simulink model "model_verification"  (R2024b)
settings: Solver=VariableStepAuto  StartTime=0.0  StopTime=10.0  RelTol=1e-3
undefined symbols (not defined in the file or in its folder): EulersEOM, IAU, juliandate, sat, WMM2020
libraries: aerolibutil x8, matrix_library x8, simulink_extras x6, sharedtransform x5, sharedutil x1, aerolibtransform2 x1, aerolibgravity2 x1
settings Model: Creator=Ameya  LastModifiedBy=Ameya

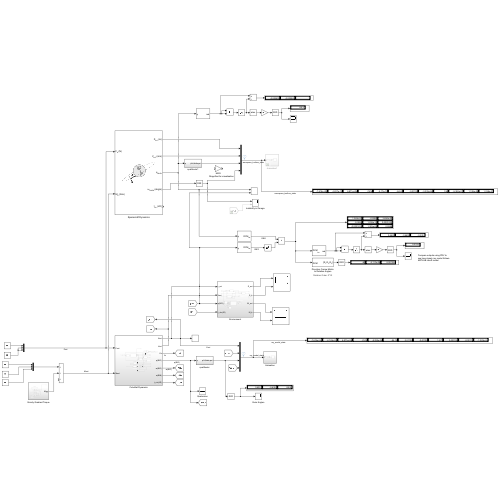
[thumbnail: Simulink's stored preview of the top-level diagram]
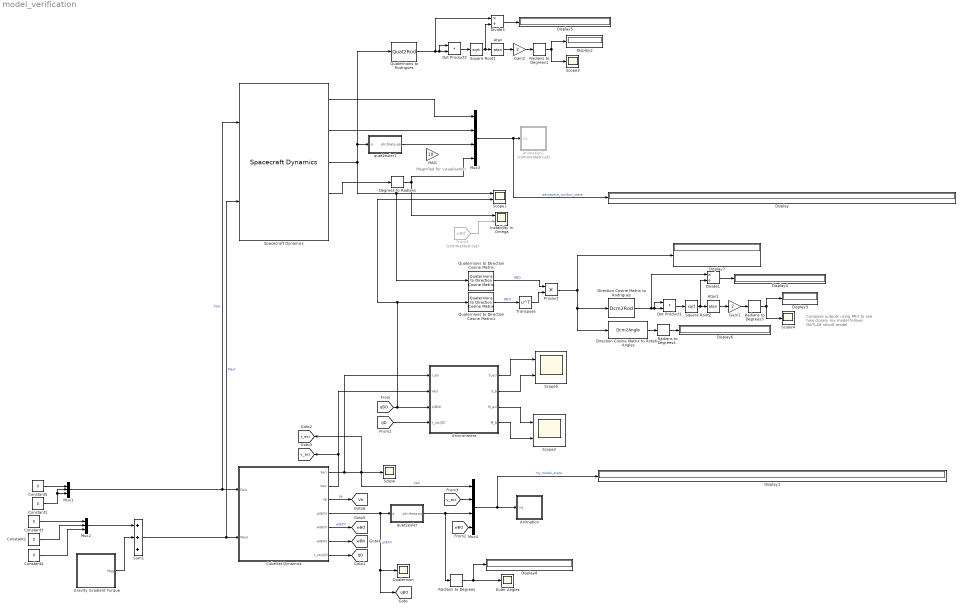
== system model_verification ==
  note: Magnified for visualisation
  note: Compare outputs using PRV to see how closely my model follows MATLAB inbuilt model
  Animation : Subsystem
  Animation1 : Subsystem  Commented=on
  Atan : Trigonometry  Operator=atan
  Atan1 : Trigonometry  Operator=atan
  Constant{1..5} (5 alike) : Constant  Value=0
  CubeSat Dynamics : Subsystem
  Degrees to Radians : simulink_extras/Transformations/Degrees to Radians
  Direction Cosine Matrix to Rotation Angles : Dcm2Angle
      settings: AttributesFormatString=Rotation Order: %<rotationOrder>
  Direction Cosine Matrix to Rodrigues : Dcm2Rod
  Display{,1..8} (9 alike) : Display
  Divide1 : Product  Inputs=*/
  Divide3 : Product  Inputs=*/
  Dot Product1 : DotProduct  OutDataTypeStr=Inherit: Inherit via internal rule
  Dot Product3 : DotProduct  OutDataTypeStr=Inherit: Inherit via internal rule
  Environment : Subsystem
  Euler Angles : Scope
  From4 : From  Commented=on  GotoTag=wBO
  Gain1 : Gain  Gain=2
  Gain2 : Gain  Gain=2
  Gravity Gradient Torque : Subsystem
  Instability in Omega : Scope  NumInputPorts=2
  MAG : Gain  Gain=10
  Mux1 : Mux  Inputs=3
  Mux2 : Mux  Inputs=3
  Mux3 : Mux
  Mux4 : Mux
  Product : Product
  Quaternion : Scope
  Quaternions to Rodrigues : Quat2Rod
  Quaternions to Direction Cosine Matrix : sharedtransform/Quaternions to  Direction Cosine Matrix  aMode=aMode
      settings: LibrarySourceBlock=|
      | aerolibtransform2/Quaternions to
      | Direction Cosine Matrix
  Quaternions to Direction Cosine Matrix1 : sharedtransform/Quaternions to  Direction Cosine Matrix  aMode=aMode
      settings: LibrarySourceBlock=|
      | aerolibtransform2/Quaternions to
      | Direction Cosine Matrix
  Radians to Degrees{,1,3..4} (4 alike) : simulink_extras/Transformations/Radians to Degrees
  Scope : Scope
  Scope1 : Scope  NumInputPorts=2
  Scope2 : Scope  NumInputPorts=2
  Scope3 : Scope
  Scope4 : Scope
  Scope5 : Scope  NumInputPorts=2
  Spacecraft Dynamics : SpacecraftDynamics  mass=sat.mass  inertia=sat.J  semiMajorAxis=sat.a  eccentricity=sat.e  inclination=rad2deg(sat.i)  raan=rad2deg(sat.RAAN)  argPeriapsis=rad2deg(sat.w)  trueAnomaly=0  attitudeFrame=LVLH  attitude=sat.quat  attitudeRate=[sat.p,sat.q,sat.r]  useGravGrad=off  gravityModel=Point-mass  useEOPs=off
  Square Root1 : Sqrt
  Square Root2 : Sqrt
  Sum1 : Sum  Inputs=+++
  Transpose : Math  Operator=transpose
  quat2euler : Subsystem
  quat2euler1 : Subsystem
  tag scope: Vb=global, qBO=global, r_eci=global, tJD=global, v_eci=global, wBN=global, wBO=global
  wires:
  Radians to Degrees/1 -> Display8/1, Euler Angles/1
  quat2euler/1(phi,theta,psi) -> Radians to Degrees/1, Mux4/3
  quat2euler1/1(phi,theta,psi) -> Mux3/3
  Gain2/1 -> Radians to Degrees1/1
  CubeSat Dynamics/4(q(B/O)) -> quat2euler/1(q), [qBO], Quaternion/1  "q(B/O)"
  Direction Cosine Matrix to Rodrigues/1 -> Divide1/1, Dot Product1/2, Dot Product1/1
  Constant5/1 -> Mux1/1
  Quaternions to Rodrigues/1 -> Divide3/1, Dot Product3/2, Dot Product3/1
  Constant3/1 -> Mux2/1
  Divide1/1 -> Display4/1
  Square Root2/1 -> Divide1/2, Atan1/1
  CubeSat Dynamics/6(w(B/N)) -> [wBN]
  Spacecraft Dynamics/4 -> Degrees to Radians/1
  Atan1/1 -> Gain1/1
  Gravity Gradient Torque/1(Mgg) -> Sum1/2
  Constant2/1 -> Mux2/2
  Dot Product1/1 -> Square Root2/1
  [qBO] -> Scope1/2, Quaternions to Direction Cosine Matrix1/1, Environment/3(q(B/O))
  Mux3/1 -> Display/1, Animation1/1(In1)  "aerospace_toolbox_state"
  [v_eci] -> Mux4/2
  Dot Product3/1 -> Square Root1/1
  Spacecraft Dynamics/1 -> Mux3/1
  Environment/1(S_eci) -> Scope5/1
  CubeSat Dynamics/1(Xeci) -> [r_eci], Scope/1, Mux4/1, Environment/1(r_eci)  "Xeci"
  Gain1/1 -> Radians to Degrees3/1
  Environment/4(M_b) -> Scope2/2
  [wBO] -> Mux4/4
  Spacecraft Dynamics/3 -> Quaternions to Direction Cosine Matrix/1, Scope1/1, quat2euler1/1(q), Quaternions to Rodrigues/1
  Constant4/1 -> Mux2/3
  Environment/2(S_b) -> Scope5/2
  Constant1/1 -> Mux1/2, Mux1/3
  Square Root1/1 -> Divide3/2, Atan/1
  Product/1 -> Direction Cosine Matrix to Rotation Angles/1, Direction Cosine Matrix to Rodrigues/1, Display7/1
  Transpose/1 -> Product/2
  Mux4/1 -> Display1/1, Animation/1(In1)  "my_model_state"
  [tJD] -> Environment/4(t_utc(JD))
  CubeSat Dynamics/5(w(B/O)) -> [wBO]  "w(B/O)"
  Radians to Degrees4/1 -> Display6/1
  CubeSat Dynamics/2(Veci) -> Environment/2(Veci), [v_eci]
  CubeSat Dynamics/3(Vb) -> [Vb]  "Vb"
  Environment/3(M_eci) -> Scope2/1
  Spacecraft Dynamics/2 -> Mux3/2
  Radians to Degrees1/1 -> Display2/1, Scope3/1
  Quaternions to Direction Cosine Matrix1/1 -> Transpose/1  "RB'O"
  Quaternions to Direction Cosine Matrix/1 -> Product/1  "RBO"
  Direction Cosine Matrix to Rotation Angles/1 -> Radians to Degrees4/1
  Atan/1 -> Gain2/1
  CubeSat Dynamics/7(t_utc(JD)) -> [tJD]
  Divide3/1 -> Display5/1
  Sum1/1 -> Spacecraft Dynamics/2, CubeSat Dynamics/2(Mext)  "Mext"
  Mux1/1 -> Spacecraft Dynamics/1, CubeSat Dynamics/1(Fext)  "Fext"
  From4/1 -> Instability in Omega/2
  Radians to Degrees3/1 -> Display3/1, Scope4/1
  Degrees to Radians/1 -> Instability in Omega/1, Mux3/4
  Mux2/1 -> Sum1/1

== system model_verification/Animation ==
  In1 : Inport
  Clock : Clock
  CubeSat Attitude Animation : MATLABFcn  MATLABFcn=drawCubeSat  OutputDimensions=0
  Mux1 : Mux  Inputs=2
  wires:
  Mux1/1 -> CubeSat Attitude Animation/1
  In1/1 -> Mux1/1
  Clock/1 -> Mux1/2  "time"

== system model_verification/Animation1 ==
  In1 : Inport
  Clock : Clock
  CubeSat Attitude Animation : MATLABFcn  MATLABFcn=drawCubeSat  OutputDimensions=0
  Mux1 : Mux  Inputs=2
  wires:
  Mux1/1 -> CubeSat Attitude Animation/1
  In1/1 -> Mux1/1
  Clock/1 -> Mux1/2  "time"

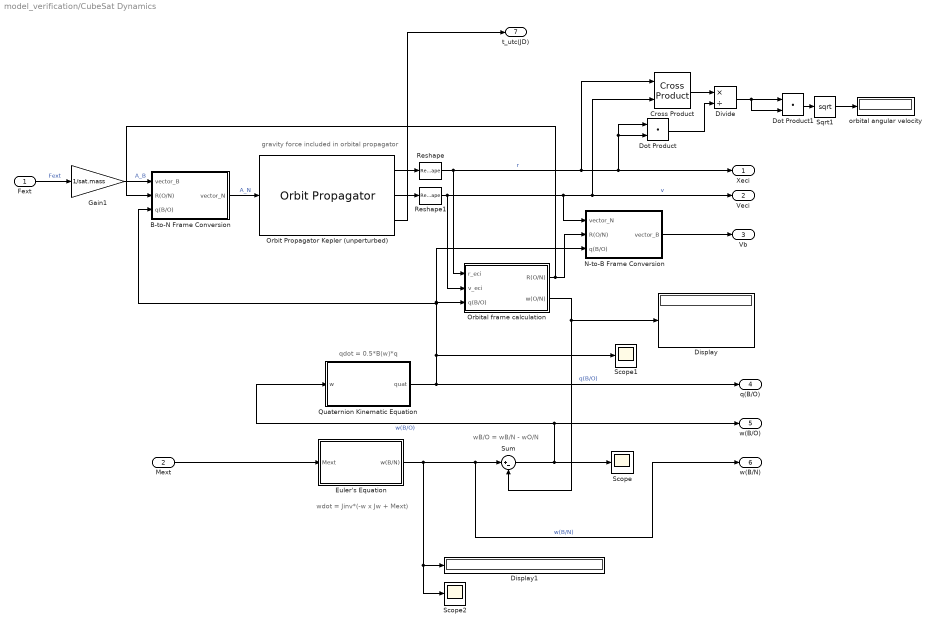
== system model_verification/CubeSat Dynamics ==
  note: wB/O = wB/N - wO/N
  note: qdot = 0.5*B(w)*q
  note: wdot = Jinv*(-w x Jw + Mext)
  note: gravity force included in orbital propagator
  Fext : Inport
  Mext : Inport  Port=2
  B-to-N Frame Conversion : Subsystem
  Cross Product : matrix_library/Cross Product
  Display : Display
  Display1 : Display
  Divide : Product  Inputs=*/
  Dot Product : DotProduct  OutDataTypeStr=Inherit: Inherit via internal rule
  Dot Product1 : DotProduct  OutDataTypeStr=Inherit: Inherit via internal rule
  Euler's Equation : Subsystem
  Gain1 : Gain  Gain=1/sat.mass
  N-to-B Frame Conversion : Subsystem
  Orbit Propagator Kepler (unperturbed) : OrbitPropagator  propagator=Numerical (high precision)  accelIn=on  startDate=juliandate(2025, 1, 1, 12, 0, 0)  semiMajorAxis=sat.a  eccentricity=sat.e  inclination=rad2deg(sat.i)  raan=rad2deg(sat.RAAN)  argPeriapsis=rad2deg(sat.w)  trueAnomaly=rad2deg(sat.ta)  inertialPosition=[3649700.0 3308200.0 -4676600.0]  inertialVelocity=[-2750.8 6666.4 2573.4]  fixedPosition=[-4142689.0 -2676864.7 -4669861.6]  fixedVelocity=[1452.7 -6720.7 2568.1]  gravityModel=Oblate ellipsoid (J2)  customR=3396200  customMu=4.305e13  customJ2=1.0826269e-03  customOmega=4.06125949e-3
  Orbital frame calculation : Subsystem
  Quaternion Kinematic Equation : Subsystem
  Reshape : Reshape  OutputDimensionality=Column vector (2-D)
  Reshape1 : Reshape  OutputDimensionality=Column vector (2-D)
  Scope : Scope
  Scope1 : Scope
  Scope2 : Scope
  Sqrt1 : Sqrt
  Sum : Sum  Inputs=|+-
  orbital angular velocity : Display
  Xeci : Outport
  Veci : Outport  Port=2
  Vb : Outport  Port=3
  q(B/O) : Outport  Port=4
  w(B/O) : Outport  Port=5
  w(B/N) : Outport  Port=6
  t_utc(JD) : Outport  Port=7
  wires:
  Mext/1 -> Euler's Equation/1(Mext)
  Euler's Equation/1(w(B/N)) -> Scope2/1, Display1/1, w(B/N)/1, Sum/1  "w(B/N)"
  Sum/1 -> w(B/O)/1, Quaternion Kinematic Equation/1(w), Scope/1  "w(B/O)"
  Orbital frame calculation/2(w(O/N)) -> Sum/2, Display/1
  Quaternion Kinematic Equation/1(quat) -> B-to-N Frame Conversion/3(q(B/O)), N-to-B Frame Conversion/3(q(B/O)), Orbital frame calculation/3(q(B/O)), Scope1/1, q(B/O)/1  "q(B/O)"
  Orbit Propagator Kepler (unperturbed)/1 -> Reshape/1
  Orbit Propagator Kepler (unperturbed)/2 -> Reshape1/1
  Reshape/1 -> Cross Product/1, Xeci/1, Dot Product/1, Dot Product/2, Orbital frame calculation/1(r_eci)  "r"
  Reshape1/1 -> N-to-B Frame Conversion/1(vector_N), Cross Product/2, Veci/1, Orbital frame calculation/2(v_eci)  "v"
  B-to-N Frame Conversion/1(vector_N) -> Orbit Propagator Kepler (unperturbed)/1  "A_N"
  Fext/1 -> Gain1/1  "Fext"
  Gain1/1 -> B-to-N Frame Conversion/1(vector_B)  "A_B"
  Orbital frame calculation/1(R(O/N)) -> B-to-N Frame Conversion/2(R(O/N)), N-to-B Frame Conversion/2(R(O/N))
  N-to-B Frame Conversion/1(vector_B) -> Vb/1
  Orbit Propagator Kepler (unperturbed)/3 -> t_utc(JD)/1
  Cross Product/1 -> Divide/1
  Dot Product/1 -> Divide/2
  Divide/1 -> Dot Product1/2, Dot Product1/1
  Dot Product1/1 -> Sqrt1/1
  Sqrt1/1 -> orbital angular velocity/1

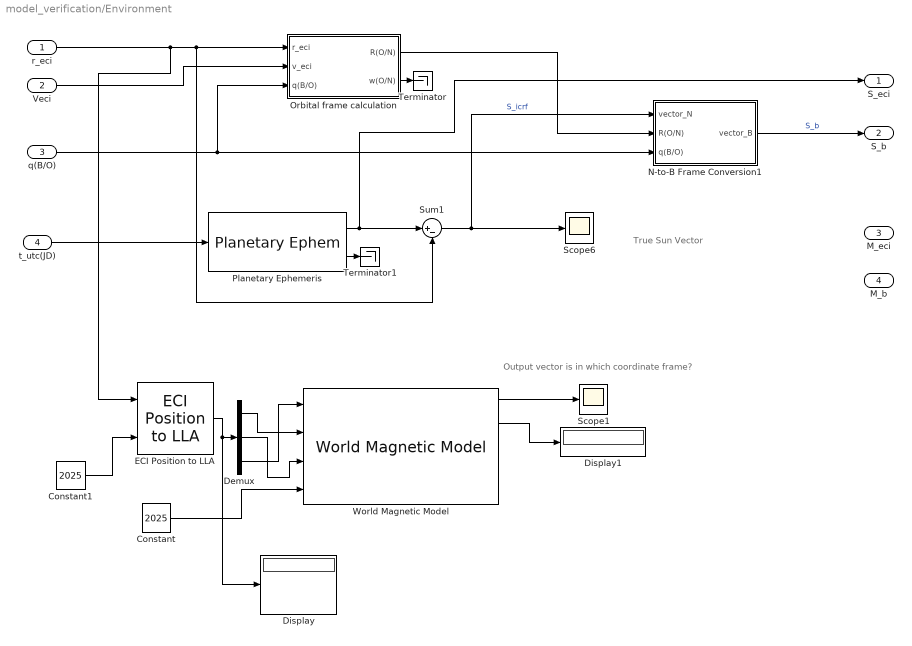
== system model_verification/Environment ==
  note: Output vector is in which coordinate frame?
  note: True Sun Vector
  r_eci : Inport
  Veci : Inport  Port=2
  q(B/O) : Inport  Port=3
  t_utc(JD) : Inport  Port=4
  Constant : Constant  Value=2025
  Constant1 : Constant  Value=2025
  Demux : Demux  Outputs=3
  Display : Display
  Display1 : Display
  ECI Position to LLA : aerolibtransform2/ECI Position to LLA  red=IAU-2000/2006  year=2025  month=January  day=1  hour=0  min=0  sec=0  deltaT=Day  errorflag=Error  extraparamflag=off  eunits=Metric (MKS)  earthmodel=WGS84  flat=1/298.257223563  eqradius=6378137
      settings: AttributesFormatString=%<red>
  N-to-B Frame Conversion1 : Subsystem
  Orbital frame calculation : Subsystem
  Planetary Ephemeris : PlanetaryEphem  target=Sun
  Scope1 : Scope
  Scope6 : Scope
  Sum1 : Sum  Inputs=|+-
  Terminator : Terminator
  Terminator1 : Terminator
  World Magnetic Model : aerolibgravity2/World Magnetic Model  model=WMM2020 (2020-2025)  customFile='WMM2020.COF'  units=Metric (MKS)  time_in=on  month=January  day=1  year=2020  action=Error  h_out=on  dec_out=on  inc_out=on  ti_out=on
  S_eci : Outport
  S_b : Outport  Port=2
  M_eci : Outport  Port=3
  M_b : Outport  Port=4
  wires:
  Orbital frame calculation/1(R(O/N)) -> N-to-B Frame Conversion1/2(R(O/N))
  Sum1/1 -> Scope6/1, N-to-B Frame Conversion1/1(vector_N)  "S_icrf"
  Planetary Ephemeris/1 -> Sum1/1, S_eci/1
  q(B/O)/1 -> N-to-B Frame Conversion1/3(q(B/O)), Orbital frame calculation/3(q(B/O))
  r_eci/1 -> ECI Position to LLA/1, Orbital frame calculation/1(r_eci), Sum1/2
  t_utc(JD)/1 -> Planetary Ephemeris/1
  N-to-B Frame Conversion1/1(vector_B) -> S_b/1  "S_b"
  Planetary Ephemeris/2 -> Terminator1/1
  Orbital frame calculation/2(w(O/N)) -> Terminator/1
  Veci/1 -> Orbital frame calculation/2(v_eci)
  Demux/3 -> World Magnetic Model/1
  Demux/1 -> World Magnetic Model/2
  Demux/2 -> World Magnetic Model/3
  World Magnetic Model/1 -> Scope1/1
  Constant1/1 -> ECI Position to LLA/2
  Constant/1 -> World Magnetic Model/4
  ECI Position to LLA/1 -> Display/1, Demux/1
  World Magnetic Model/2 -> Display1/1

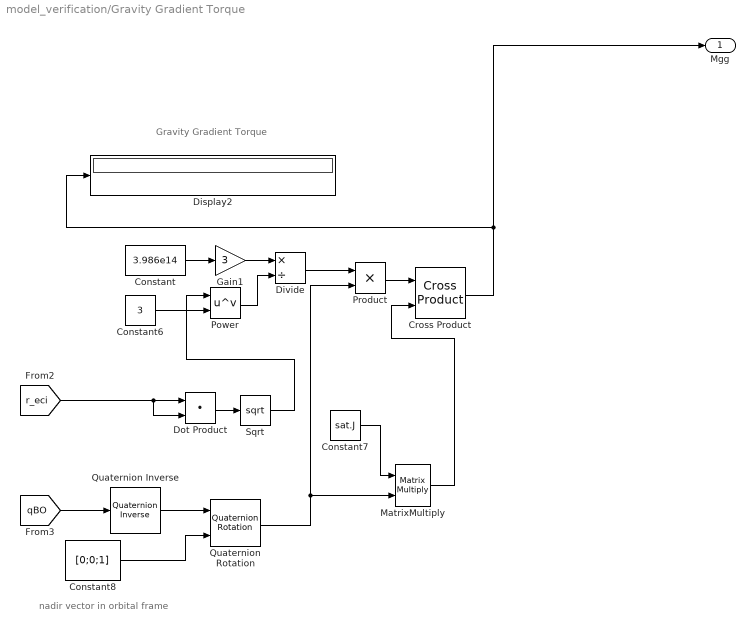
== system model_verification/Gravity Gradient Torque ==
  note: Gravity Gradient Torque
  note: nadir vector in orbital frame
  Constant : Constant  Value=3.986e14
  Constant6 : Constant  Value=3
  Constant7 : Constant  Value=sat.J
  Constant8 : Constant  Value=[0;0;1]
  Cross Product : matrix_library/Cross Product
  Display2 : Display
  Divide : Product  Inputs=*/
  Dot Product : DotProduct  OutDataTypeStr=Inherit: Inherit via internal rule
  Gain1 : Gain  Gain=3
  MatrixMultiply : Product  Multiplication=Matrix(*)
  Power : Math  Operator=pow
  Product : Product
  Quaternion Inverse : aerolibutil/Quaternion Inverse
  Quaternion Rotation : aerolibutil/Quaternion Rotation
  Sqrt : Sqrt
  Mgg : Outport
  wires:
  Power/1 -> Divide/2
  Cross Product/1 -> Mgg/1, Display2/1
  MatrixMultiply/1 -> Cross Product/2
  Quaternion Inverse/1 -> Quaternion Rotation/1
  [qBO] -> Quaternion Inverse/1
  Sqrt/1 -> Power/1
  [r_eci] -> Dot Product/2, Dot Product/1
  Product/1 -> Cross Product/1
  Constant6/1 -> Power/2
  Dot Product/1 -> Sqrt/1
  Divide/1 -> Product/1
  Quaternion Rotation/1 -> Product/2, MatrixMultiply/2
  Gain1/1 -> Divide/1
  Constant/1 -> Gain1/1
  Constant8/1 -> Quaternion Rotation/2
  Constant7/1 -> MatrixMultiply/1

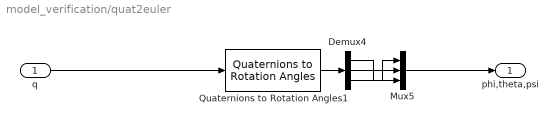
== system model_verification/quat2euler ==
  q : Inport
  Demux4 : Demux  Outputs=3
  Mux5 : Mux  Inputs=3
  Quaternions to Rotation Angles1 : sharedtransform/Quaternions to Rotation Angles  rotationOrder=ZYX  aMode=aMode
  phi,theta,psi : Outport
  wires:
  Quaternions to Rotation Angles1/1 -> Demux4/1
  Demux4/3 -> Mux5/1
  Demux4/2 -> Mux5/2
  Demux4/1 -> Mux5/3
  q/1 -> Quaternions to Rotation Angles1/1
  Mux5/1 -> phi,theta,psi/1

== system model_verification/quat2euler1 ==
  q : Inport
  Demux4 : Demux  Outputs=3
  Mux5 : Mux  Inputs=3
  Quaternions to Rotation Angles1 : sharedtransform/Quaternions to Rotation Angles  rotationOrder=ZYX  aMode=aMode
  phi,theta,psi : Outport
  wires:
  Quaternions to Rotation Angles1/1 -> Demux4/1
  Demux4/3 -> Mux5/1
  Demux4/2 -> Mux5/2
  Demux4/1 -> Mux5/3
  q/1 -> Quaternions to Rotation Angles1/1
  Mux5/1 -> phi,theta,psi/1

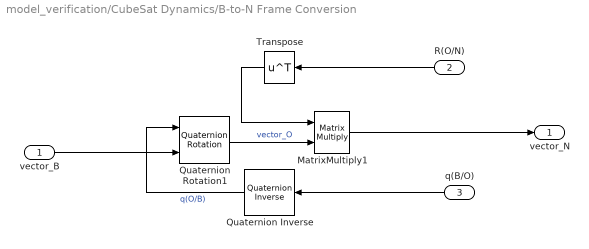
== system model_verification/CubeSat Dynamics/B-to-N Frame Conversion ==
  vector_B : Inport
  R(O/N) : Inport  Port=2
  q(B/O) : Inport  Port=3
  MatrixMultiply1 : Product  Multiplication=Matrix(*)
  Quaternion Inverse : aerolibutil/Quaternion Inverse
  Quaternion Rotation1 : aerolibutil/Quaternion Rotation
  Transpose : Math  Operator=transpose
  vector_N : Outport
  wires:
  Transpose/1 -> MatrixMultiply1/1
  MatrixMultiply1/1 -> vector_N/1
  R(O/N)/1 -> Transpose/1
  Quaternion Inverse/1 -> Quaternion Rotation1/1  "q(O/B)"
  Quaternion Rotation1/1 -> MatrixMultiply1/2  "vector_O"
  q(B/O)/1 -> Quaternion Inverse/1
  vector_B/1 -> Quaternion Rotation1/2

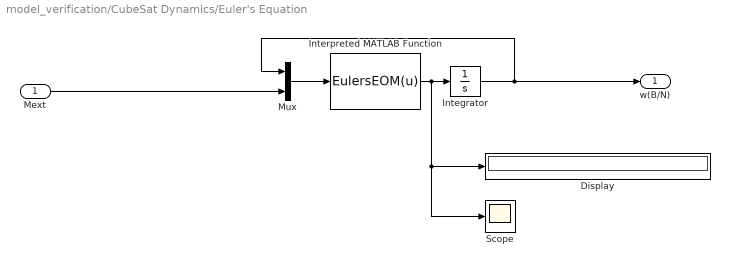
== system model_verification/CubeSat Dynamics/Euler's Equation ==
  Mext : Inport
  Display : Display
  Integrator : Integrator  InitialCondition=sat.omegaBN
  Interpreted MATLAB Function : MATLABFcn  MATLABFcn=EulersEOM(u)  OutputDimensions=3
  Mux : Mux  Inputs=2
  Scope : Scope
  w(B/N) : Outport
  wires:
  Integrator/1 -> w(B/N)/1, Mux/1
  Interpreted MATLAB Function/1 -> Display/1, Scope/1, Integrator/1
  Mext/1 -> Mux/2
  Mux/1 -> Interpreted MATLAB Function/1

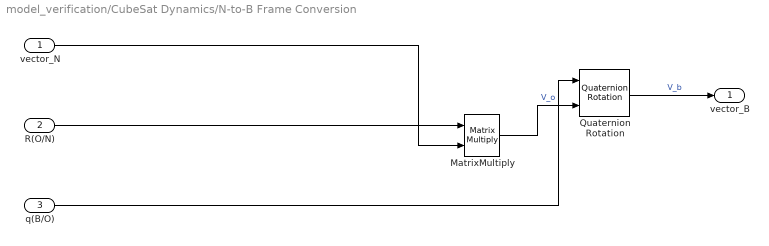
== system model_verification/CubeSat Dynamics/N-to-B Frame Conversion ==
  vector_N : Inport
  R(O/N) : Inport  Port=2
  q(B/O) : Inport  Port=3
  MatrixMultiply : Product  Multiplication=Matrix(*)
  Quaternion Rotation : aerolibutil/Quaternion Rotation
  vector_B : Outport
  wires:
  MatrixMultiply/1 -> Quaternion Rotation/2  "V_o"
  Quaternion Rotation/1 -> vector_B/1  "V_b"
  R(O/N)/1 -> MatrixMultiply/1
  vector_N/1 -> MatrixMultiply/2
  q(B/O)/1 -> Quaternion Rotation/1

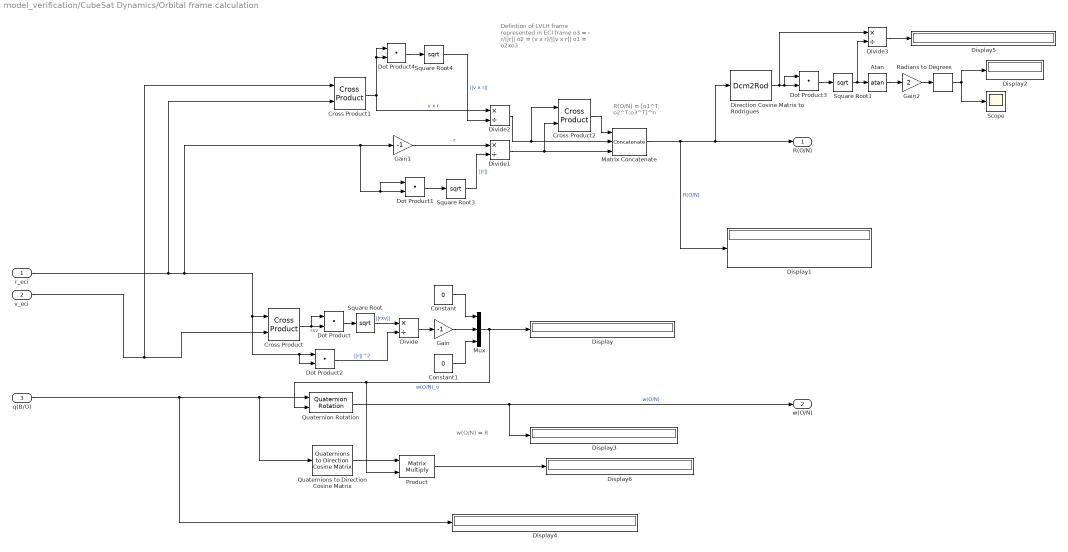
== system model_verification/CubeSat Dynamics/Orbital frame calculation ==
  note: w(O/N) = R
  note: R(O/N) = [o1^T; o2^T;o3^T]^n
  note: Defintion of LVLH frame
      | represented in ECI frame
      | o3 = - r/||r||
      | o2 = (v x r)/||v x r||
      | o1 = o2xo3
  r_eci : Inport
  v_eci : Inport  Port=2
  q(B/O) : Inport  Port=3
  Atan : Trigonometry  Operator=atan
  Constant : Constant  Value=0
  Constant1 : Constant  Value=0
  Cross Product : matrix_library/Cross Product
  Cross Product1 : matrix_library/Cross Product
  Cross Product2 : matrix_library/Cross Product
  Direction Cosine Matrix to Rodrigues : Dcm2Rod
  Display{,1..6} (7 alike) : Display
  Divide{,1..3} (4 alike) : Product  Inputs=*/
  Dot Product{,1..4} (5 alike) : DotProduct  OutDataTypeStr=Inherit: Inherit via internal rule
  Gain : Gain  Gain=-1
  Gain1 : Gain  Gain=-1
  Gain2 : Gain  Gain=2
  Matrix Concatenate : Concatenate  NumInputs=3  Mode=Multidimensional array  ConcatenateDimension=2
  Mux : Mux  Inputs=3
  Product : Product  Multiplication=Matrix(*)
  Quaternion Rotation : aerolibutil/Quaternion Rotation
  Quaternions to Direction Cosine Matrix : sharedtransform/Quaternions to  Direction Cosine Matrix  aMode=aMode
  Radians to Degrees : simulink_extras/Transformations/Radians to Degrees
  Scope : Scope
  Square Root{,1,3..4} (4 alike) : Sqrt
  R(O/N) : Outport
  w(O/N) : Outport  Port=2
  wires:
  Constant1/1 -> Mux/3
  Dot Product2/1 -> Divide/2  "||r||^2"
  Gain/1 -> Mux/2
  q(B/O)/1 -> Quaternion Rotation/1, Quaternions to Direction Cosine Matrix/1, Display4/1
  Quaternion Rotation/1 -> w(O/N)/1, Display3/1  "w(O/N)"
  Cross Product/1 -> Dot Product/1, Dot Product/2  "rxv"
  Dot Product/1 -> Square Root/1
  Divide/1 -> Gain/1
  Square Root/1 -> Divide/1  "||rxv||"
  Mux/1 -> Product/2, Quaternion Rotation/2, Display/1  "w(O/N)_o"
  Constant/1 -> Mux/1
  Cross Product2/1 -> Matrix Concatenate/1
  Divide2/1 -> Cross Product2/1, Matrix Concatenate/2
  Cross Product1/1 -> Dot Product4/2, Dot Product4/1, Divide2/1  "v x r"
  r_eci/1 -> Cross Product1/2, Dot Product1/1, Dot Product1/2, Gain1/1, Dot Product2/2, Dot Product2/1, Cross Product/1
  Gain1/1 -> Divide1/1  "- r"
  Square Root3/1 -> Divide1/2  "||r||"
  Square Root4/1 -> Divide2/2  "||v x r||"
  Dot Product1/1 -> Square Root3/1
  v_eci/1 -> Cross Product1/1, Cross Product/2
  Matrix Concatenate/1 -> R(O/N)/1, Direction Cosine Matrix to Rodrigues/1, Display1/1  "R(O/N)"
  Divide1/1 -> Cross Product2/2, Matrix Concatenate/3
  Dot Product4/1 -> Square Root4/1
  Direction Cosine Matrix to Rodrigues/1 -> Divide3/1, Dot Product3/2, Dot Product3/1
  Dot Product3/1 -> Square Root1/1
  Square Root1/1 -> Divide3/2, Atan/1
  Radians to Degrees/1 -> Display2/1, Scope/1
  Divide3/1 -> Display5/1
  Atan/1 -> Gain2/1
  Gain2/1 -> Radians to Degrees/1
  Quaternions to Direction Cosine Matrix/1 -> Product/1
  Product/1 -> Display6/1

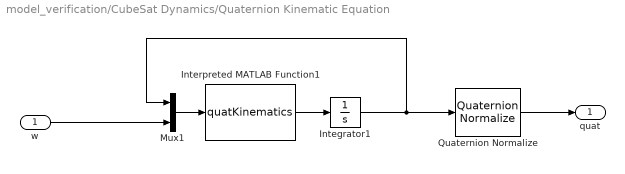
== system model_verification/CubeSat Dynamics/Quaternion Kinematic Equation ==
  w : Inport
  Integrator1 : Integrator  InitialCondition=sat.quat
  Interpreted MATLAB Function1 : MATLABFcn  MATLABFcn=quatKinematics  OutputDimensions=4
  Mux1 : Mux  Inputs=2
  Quaternion Normalize : sharedutil/Quaternion Normalize  aMode=aMode
  quat : Outport
  wires:
  Mux1/1 -> Interpreted MATLAB Function1/1
  Integrator1/1 -> Quaternion Normalize/1, Mux1/1
  Interpreted MATLAB Function1/1 -> Integrator1/1
  w/1 -> Mux1/2
  Quaternion Normalize/1 -> quat/1

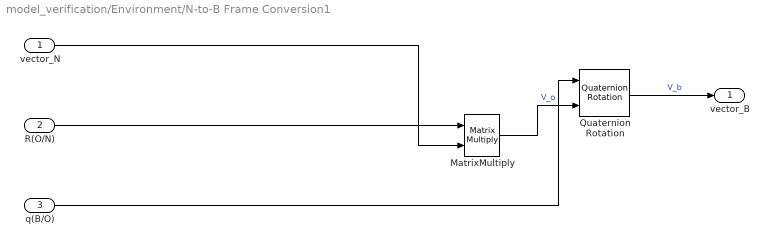
== system model_verification/Environment/N-to-B Frame Conversion1 ==
  vector_N : Inport
  R(O/N) : Inport  Port=2
  q(B/O) : Inport  Port=3
  MatrixMultiply : Product  Multiplication=Matrix(*)
  Quaternion Rotation : aerolibutil/Quaternion Rotation
  vector_B : Outport
  wires:
  MatrixMultiply/1 -> Quaternion Rotation/2  "V_o"
  Quaternion Rotation/1 -> vector_B/1  "V_b"
  R(O/N)/1 -> MatrixMultiply/1
  vector_N/1 -> MatrixMultiply/2
  q(B/O)/1 -> Quaternion Rotation/1

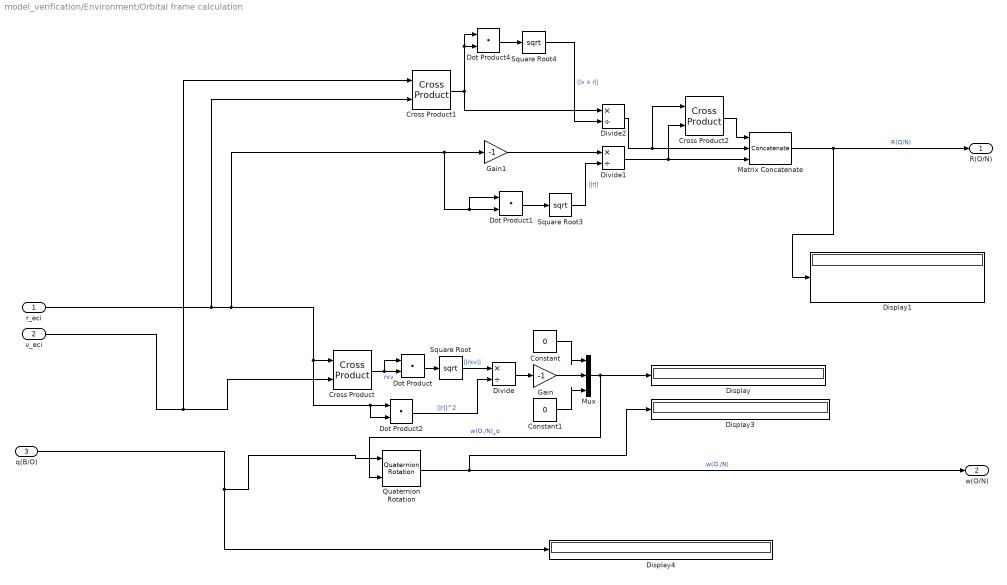
== system model_verification/Environment/Orbital frame calculation ==
  r_eci : Inport
  v_eci : Inport  Port=2
  q(B/O) : Inport  Port=3
  Constant : Constant  Value=0
  Constant1 : Constant  Value=0
  Cross Product : matrix_library/Cross Product
  Cross Product1 : matrix_library/Cross Product
  Cross Product2 : matrix_library/Cross Product
  Display{,1,3..4} (4 alike) : Display
  Divide : Product  Inputs=*/
  Divide1 : Product  Inputs=*/
  Divide2 : Product  Inputs=*/
  Dot Product{,1..2,4} (4 alike) : DotProduct  OutDataTypeStr=Inherit: Inherit via internal rule
  Gain : Gain  Gain=-1
  Gain1 : Gain  Gain=-1
  Matrix Concatenate : Concatenate  NumInputs=3  Mode=Multidimensional array  ConcatenateDimension=2
  Mux : Mux  Inputs=3
  Quaternion Rotation : aerolibutil/Quaternion Rotation
  Square Root : Sqrt
  Square Root3 : Sqrt
  Square Root4 : Sqrt
  R(O/N) : Outport
  w(O/N) : Outport  Port=2
  wires:
  Constant1/1 -> Mux/3
  Dot Product2/1 -> Divide/2  "||r||^2"
  Gain/1 -> Mux/2
  q(B/O)/1 -> Display4/1, Quaternion Rotation/1
  Quaternion Rotation/1 -> Display3/1, w(O/N)/1  "w(O./N)"
  Cross Product/1 -> Dot Product/1, Dot Product/2  "rxv"
  Dot Product/1 -> Square Root/1
  Divide/1 -> Gain/1
  Square Root/1 -> Divide/1  "||rxv||"
  Mux/1 -> Quaternion Rotation/2, Display/1  "w(O./N)_o"
  Constant/1 -> Mux/1
  Cross Product2/1 -> Matrix Concatenate/1
  Divide2/1 -> Cross Product2/1, Matrix Concatenate/2
  Cross Product1/1 -> Dot Product4/2, Dot Product4/1, Divide2/1
  r_eci/1 -> Cross Product1/2, Dot Product1/1, Dot Product1/2, Gain1/1, Dot Product2/2, Dot Product2/1, Cross Product/1
  Gain1/1 -> Divide1/1
  Square Root3/1 -> Divide1/2  "||r||"
  Square Root4/1 -> Divide2/2  "||v x r||"
  Dot Product1/1 -> Square Root3/1
  v_eci/1 -> Cross Product1/1, Cross Product/2
  Matrix Concatenate/1 -> R(O/N)/1, Display1/1  "R(O/N)"
  Divide1/1 -> Cross Product2/2, Matrix Concatenate/3
  Dot Product4/1 -> Square Root4/1
